simulink model "Vjezba2"  (R2023b)
settings: Solver=ode1  StartTime=0.0  StopTime=simulationTime  FixedStep=sampleTime  RelTol=1e-3  EnableMultiTasking=on
InitFcn:
  | cd(fileparts(which(gcs)))
  | 
  | run ./InitModel.m;
StopFcn:
  | run ./DrawPath.m;
values from neighbouring files (symbols this model uses):
  sampleTime = 1e-2    (= 0.01)    [InitModel.m]
  SWA = 3    [InitModel.m]
  vx0 = 200    [InitModel.m]
undefined symbols (not defined in the file or in its folder): vehicleData
libraries: simulink_extras x1
settings Model: Creator=arikera  LastModifiedBy=lvuke
settings SolverCC: AlgebraicLoopSolver=TrustRegion
settings DataIOCC: LimitDataPoints=on  SaveFormat=Array  SignalLoggingSaveFormat=ModelDataLogs  ReturnWorkspaceOutputs=off
settings OptimizationCC: ExpressionDepthLimit=2147483647  LifeSpan=inf
settings DebuggingCC: UnderspecifiedInitializationDetection=Classic  MergeDetectMultiDrivingBlocksExec=none  SolverPrmCheckMsg=warning  FcnCallInpInsideContextMsg=warning  UnconnectedInputMsg=warning  UnconnectedOutputMsg=warning  UnconnectedLineMsg=warning  AllowSymbolicDim=off  StateNameClashWarn=warning  SFUnexpectedBacktrackingDiag=warning  SFNoUnconditionalDefaultTransitionDiag=warning  SFExecutionAtInitializationDiag=none  ArithmeticOperatorsInVariantConditions=warning
settings HardwareCC: ProdBitPerPointer=32  ProdBitPerSizeT=32  ProdBitPerPtrDiffT=32  ProdLargestAtomicFloat=None  ProdIntDivRoundTo=Undefined  ProdEndianess=Unspecified  ProdWordSize=32  ProdHWDeviceType=32-bit Generic
settings ModelReferenceCC: EnableRefExpFcnMdlSchedulingChecks=on  PropagateSignalLabelsOutOfModel=off
settings SFSimCC: SimUseLocalCustomCode=off  CustomCodeUndefinedFunction=UseInterfaceOnly
settings RTWCC: RTWUseLocalCustomCode=off
settings CodeAppCC: StateflowObjectComments=on
settings GRTTargetCC: TargetLangStandard=C89/C90 (ANSI)  CombineOutputUpdateFcns=off  GRTInterface=on
settings ConfigComp: CovMetricSettings=dw  CovSaveCumulativeToWorkspaceVar=on  CovSaveSingleToWorkspaceVar=on  CovExternalEMLEnable=off  CovSFcnEnable=off

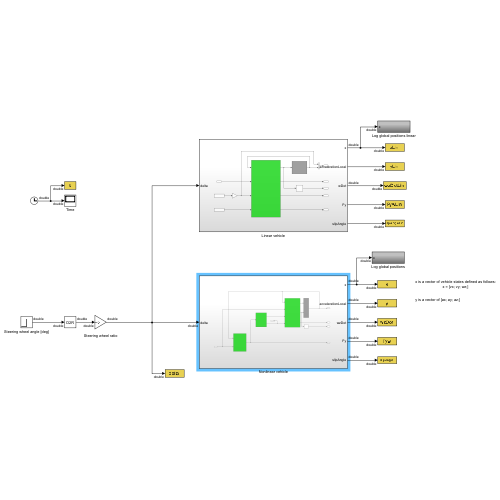
[thumbnail: Simulink's stored preview of the top-level diagram]
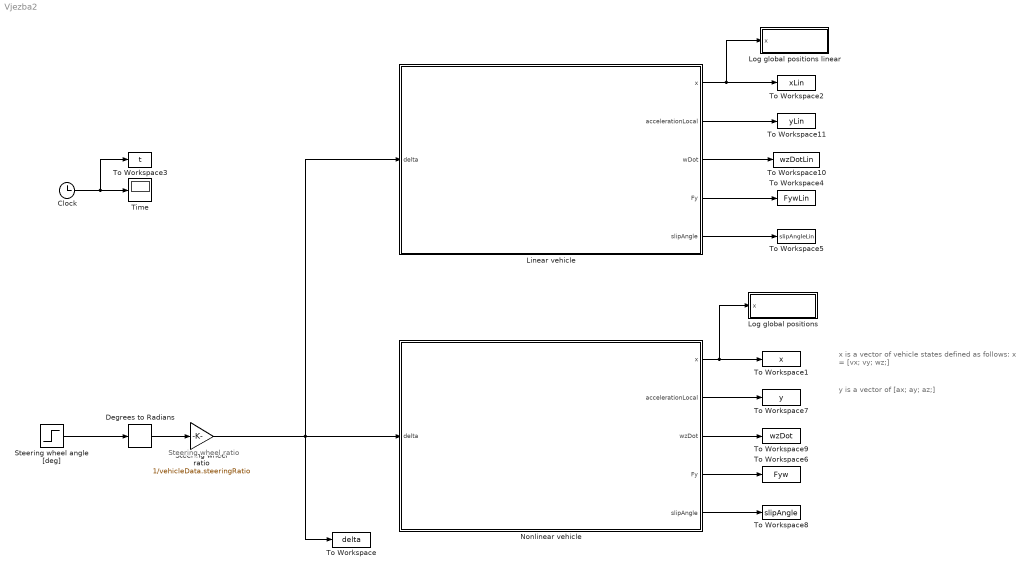
== system Vjezba2 ==
  note: Steering wheel ratio
  note: x is a vector of vehicle states defined as follows:
      | x = [vx; vy; wz;]
  note: y is a vector of [ax; ay; az;]
  Clock : Clock
  Degrees to Radians : simulink_extras/Transformations/Degrees to Radians
  Linear vehicle : Subsystem
  Log global positions : Subsystem
  Log global positions linear : Subsystem
  Nonlinear vehicle : Subsystem
  Steering wheel angle [deg] : Step  Time=3  After=SWA  SampleTime=0
  Steering wheel ratio : Gain  Gain=1/vehicleData.steeringRatio
  Time : Display
  To Workspace : ToWorkspace  VariableName=delta  SampleTime=sampleTime
  To Workspace1 : ToWorkspace  VariableName=x  SampleTime=sampleTime
  To Workspace10 : ToWorkspace  VariableName=wzDotLin  SampleTime=sampleTime
  To Workspace11 : ToWorkspace  VariableName=yLin  SampleTime=sampleTime
  To Workspace2 : ToWorkspace  VariableName=xLin  SampleTime=sampleTime
  To Workspace3 : ToWorkspace  VariableName=t  SampleTime=sampleTime
  To Workspace4 : ToWorkspace  VariableName=FywLin  SampleTime=sampleTime
  To Workspace5 : ToWorkspace  VariableName=slipAngleLin  SampleTime=sampleTime
  To Workspace6 : ToWorkspace  VariableName=Fyw  SampleTime=sampleTime
  To Workspace7 : ToWorkspace  VariableName=y  SampleTime=sampleTime
  To Workspace8 : ToWorkspace  VariableName=slipAngle  SampleTime=sampleTime
  To Workspace9 : ToWorkspace  VariableName=wzDot  SampleTime=sampleTime
  wires:
  Clock/1 -> To Workspace3/1, Time/1
  Steering wheel angle [deg]/1 -> Degrees to Radians/1
  Nonlinear vehicle/1(x) -> Log global positions/1(x), To Workspace1/1
  Nonlinear vehicle/2(accelerationLocal) -> To Workspace7/1
  Nonlinear vehicle/3(wzDot) -> To Workspace9/1
  Nonlinear vehicle/4(Fy) -> To Workspace6/1
  Nonlinear vehicle/5(slipAngle) -> To Workspace8/1
  Linear vehicle/1(x) -> Log global positions linear/1(x), To Workspace2/1
  Linear vehicle/3(wDot) -> To Workspace10/1
  Steering wheel ratio/1 -> Linear vehicle/1(delta), To Workspace/1, Nonlinear vehicle/1(delta)
  Linear vehicle/2(accelerationLocal) -> To Workspace11/1
  Degrees to Radians/1 -> Steering wheel ratio/1
  Linear vehicle/4(Fy) -> To Workspace4/1
  Linear vehicle/5(slipAngle) -> To Workspace5/1

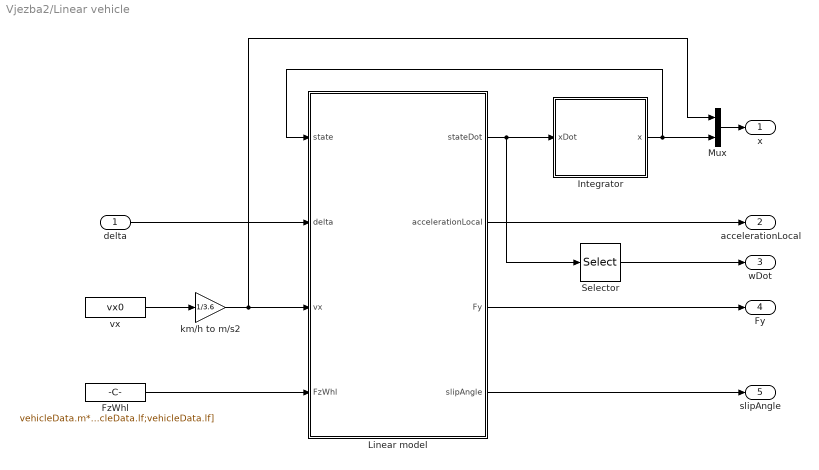
== system Vjezba2/Linear vehicle ==
  delta : Inport
  FzWhl : Constant  Value=vehicleData.m*vehicleData.g/(2*vehicleData.L)*[vehicleData.lr;vehicleData.lr;vehicleData.lf;vehicleData.lf]  SampleTime=0
  Integrator : Subsystem
  Linear model : MATLAB Function  TreatAsAtomicUnit=on
  Mux : Mux  Inputs=2
  Selector : Selector  InputPortWidth=2  IndexOptions=Index vector (dialog)  Indices=[2]  OutputSizes=1
  km/h to m/s2 : Gain  Gain=1/3.6
  vx : Constant  Value=vx0  SampleTime=0
  x : Outport  VectorParamsAs1DForOutWhenUnconnected=off
  accelerationLocal : Outport  Port=2
  wDot : Outport  Port=3  VectorParamsAs1DForOutWhenUnconnected=off
  Fy : Outport  Port=4  VectorParamsAs1DForOutWhenUnconnected=off
  slipAngle : Outport  Port=5  VectorParamsAs1DForOutWhenUnconnected=off
  wires:
  FzWhl/1 -> Linear model/4(FzWhl)
  Linear model/1(stateDot) -> Selector/1, Integrator/1(xDot)
  Integrator/1(x) -> Mux/2, Linear model/1(state)
  delta/1 -> Linear model/2(delta)
  Selector/1 -> wDot/1
  Mux/1 -> x/1
  vx/1 -> km/h to m/s2/1
  km/h to m/s2/1 -> Mux/1, Linear model/3(vx)
  Linear model/2(accelerationLocal) -> accelerationLocal/1
  Linear model/4(slipAngle) -> slipAngle/1
  Linear model/3(Fy) -> Fy/1

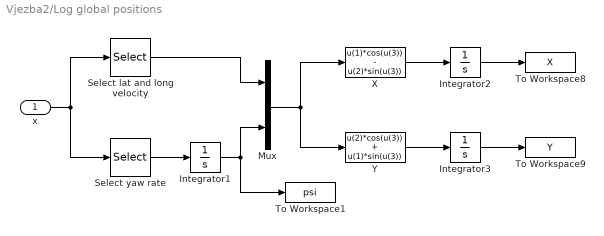
== system Vjezba2/Log global positions ==
  x : Inport
  Integrator1 : Integrator
  Integrator2 : Integrator
  Integrator3 : Integrator
  Mux : Mux  Inputs=2
  Select yaw rate : Selector  InputPortWidth=3  IndexOptions=Index vector (dialog)  Indices=3  OutputSizes=1
  Select lat and long velocity : Selector  InputPortWidth=3  IndexOptions=Index vector (dialog)  Indices=[1 2]  OutputSizes=1
  To Workspace1 : ToWorkspace  VariableName=psi  SampleTime=sampleTime
  To Workspace8 : ToWorkspace  VariableName=X  SampleTime=sampleTime
  To Workspace9 : ToWorkspace  VariableName=Y  SampleTime=sampleTime
  X : Fcn  Expr=u(1)*cos(u(3)) - u(2)*sin(u(3))
  Y : Fcn  Expr=u(2)*cos(u(3)) + u(1)*sin(u(3))
  wires:
  Select yaw rate/1 -> Integrator1/1
  Select lat and long velocity/1 -> Mux/1
  Integrator1/1 -> Mux/2, To Workspace1/1
  Mux/1 -> X/1, Y/1
  X/1 -> Integrator2/1
  Y/1 -> Integrator3/1
  x/1 -> Select yaw rate/1, Select lat and long velocity/1
  Integrator2/1 -> To Workspace8/1
  Integrator3/1 -> To Workspace9/1

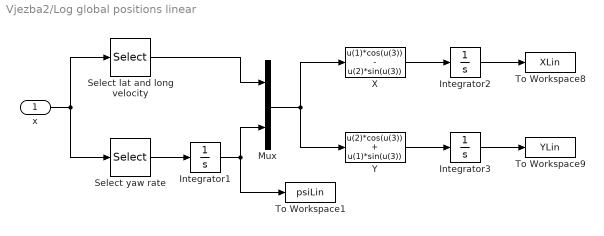
== system Vjezba2/Log global positions linear ==
  x : Inport
  Integrator1 : Integrator
  Integrator2 : Integrator
  Integrator3 : Integrator
  Mux : Mux  Inputs=2
  Select yaw rate : Selector  InputPortWidth=3  IndexOptions=Index vector (dialog)  Indices=3  OutputSizes=1
  Select lat and long velocity : Selector  InputPortWidth=3  IndexOptions=Index vector (dialog)  Indices=[1 2]  OutputSizes=1
  To Workspace1 : ToWorkspace  VariableName=psiLin  SampleTime=sampleTime
  To Workspace8 : ToWorkspace  VariableName=XLin  SampleTime=sampleTime
  To Workspace9 : ToWorkspace  VariableName=YLin  SampleTime=sampleTime
  X : Fcn  Expr=u(1)*cos(u(3)) - u(2)*sin(u(3))
  Y : Fcn  Expr=u(2)*cos(u(3)) + u(1)*sin(u(3))
  wires:
  Select yaw rate/1 -> Integrator1/1
  Select lat and long velocity/1 -> Mux/1
  Integrator1/1 -> Mux/2, To Workspace1/1
  Mux/1 -> X/1, Y/1
  X/1 -> Integrator2/1
  Y/1 -> Integrator3/1
  x/1 -> Select yaw rate/1, Select lat and long velocity/1
  Integrator2/1 -> To Workspace8/1
  Integrator3/1 -> To Workspace9/1

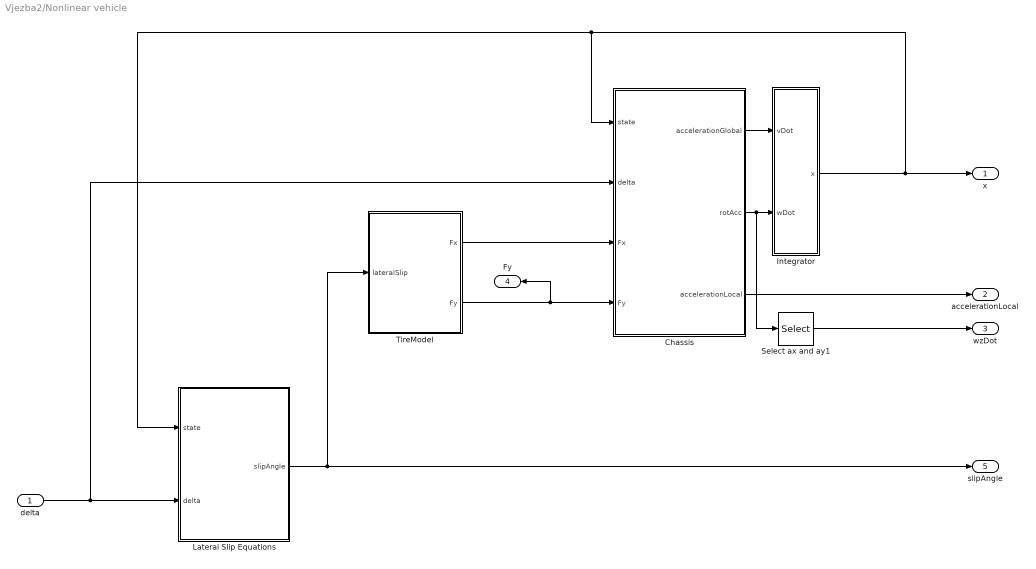
== system Vjezba2/Nonlinear vehicle ==
  delta : Inport
  Chassis : MATLAB Function  TreatAsAtomicUnit=on
  Integrator : Subsystem
  Lateral Slip Equations : MATLAB Function  TreatAsAtomicUnit=on
  Select ax and ay1 : Selector  InputPortWidth=3  IndexOptions=Index vector (dialog)  Indices=[3]  OutputSizes=1
  TireModel : Subsystem
  x : Outport
  accelerationLocal : Outport  Port=2
  wzDot : Outport  Port=3
  Fy : Outport  Port=4
  slipAngle : Outport  Port=5
  wires:
  Chassis/2(rotAcc) -> Select ax and ay1/1, Integrator/2(wDot)
  Chassis/1(accelerationGlobal) -> Integrator/1(vDot)
  delta/1 -> Lateral Slip Equations/2(delta), Chassis/2(delta)
  TireModel/2(Fy) -> Fy/1, Chassis/4(Fy)
  TireModel/1(Fx) -> Chassis/3(Fx)
  Lateral Slip Equations/1(slipAngle) -> slipAngle/1, TireModel/1(lateralSlip)
  Chassis/3(accelerationLocal) -> accelerationLocal/1
  Integrator/1(x) -> Chassis/1(state), Lateral Slip Equations/1(state), x/1
  Select ax and ay1/1 -> wzDot/1

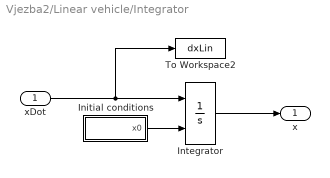
== system Vjezba2/Linear vehicle/Integrator ==
  xDot : Inport
  Initial conditions : Subsystem  mask(x0){v0=0, r0=0}
      mask prompts: v0 "Lateral velocity [km/h]"; r0 "Yaw rate [deg/s]"
      mask help: Initial conditions for the simulation
      mask Help:
      | Sets the initial condition for the simulation.
      | 
      | This is a rather simple block that has been made for assignments in the Vehicle Dynamics course (MMF062) at Chalmers since most students enrolled in this course have no prior experience in Simulink.
      | 
      | This block is equivalent to a constant source block with the vector '[u0, v0, r0, ax0, ay0, rDot0]' as the input, where the parameters are as follows:
      | 
      | u0  - Initial longitudinal velocity
      | v0  - Initial lateral velocity
      | r0  - Initial yaw rate
      | 
      | All the parameters are in SI units.
  Integrator : Integrator  InitialConditionSource=external
  To Workspace2 : ToWorkspace  VariableName=dxLin  SampleTime=sampleTime
  x : Outport  VectorParamsAs1DForOutWhenUnconnected=off
  wires:
  Initial conditions/1(x0) -> Integrator/2
  Integrator/1 -> x/1
  xDot/1 -> To Workspace2/1, Integrator/1

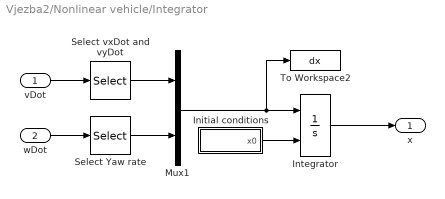
== system Vjezba2/Nonlinear vehicle/Integrator ==
  vDot : Inport
  wDot : Inport  Port=2
  Initial conditions : Subsystem  mask(x0){u0=vx0, v0=0, r0=0}
      mask prompts: u0 "Longitudinal velocity [km/h]"; v0 "Lateral velocity [km/h]"; r0 "Yaw rate [deg/s]"
      mask help: Initial conditions for the simulation
      mask Help:
      | Sets the initial condition for the simulation.
      | 
      | This is a rather simple block that has been made for assignments in the Vehicle Dynamics course (MMF062) at Chalmers since most students enrolled in this course have no prior experience in Simulink.
      | 
      | This block is equivalent to a constant source block with the vector '[u0, v0, r0, ax0, ay0, rDot0]' as the input, where the parameters are as follows:
      | 
      | u0  - Initial longitudinal velocity
      | v0  - Initial lateral velocity
      | r0  - Initial yaw rate
      | 
      | All the parameters are in SI units.
  Integrator : Integrator  InitialConditionSource=external
  Mux1 : Mux  Inputs=2
  Select Yaw rate : Selector  InputPortWidth=3  IndexOptions=Index vector (dialog)  Indices=[3]  OutputSizes=1
  Select vxDot and vyDot : Selector  InputPortWidth=3  IndexOptions=Index vector (dialog)  Indices=[1 2]  OutputSizes=1
  To Workspace2 : ToWorkspace  VariableName=dx  SampleTime=sampleTime
  x : Outport  VectorParamsAs1DForOutWhenUnconnected=off
  wires:
  Select Yaw rate/1 -> Mux1/2
  wDot/1 -> Select Yaw rate/1
  Select vxDot and vyDot/1 -> Mux1/1
  vDot/1 -> Select vxDot and vyDot/1
  Mux1/1 -> To Workspace2/1, Integrator/1
  Initial conditions/1(x0) -> Integrator/2
  Integrator/1 -> x/1

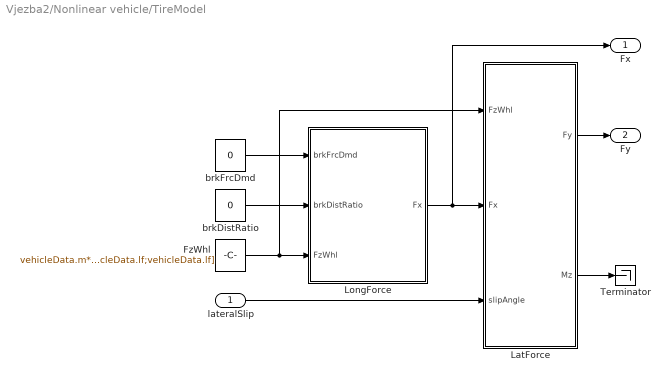
== system Vjezba2/Nonlinear vehicle/TireModel ==
  lateralSlip : Inport
  FzWhl : Constant  Value=vehicleData.m*vehicleData.g/(2*vehicleData.L)*[vehicleData.lr;vehicleData.lr;vehicleData.lf;vehicleData.lf]  SampleTime=0
  LatForce : MATLAB Function  TreatAsAtomicUnit=on
  LongForce : MATLAB Function  TreatAsAtomicUnit=on
  Terminator : Terminator
  brkDistRatio : Constant  Value=0  SampleTime=0
  brkFrcDmd : Constant  Value=0  SampleTime=0
  Fx : Outport  VectorParamsAs1DForOutWhenUnconnected=off
  Fy : Outport  Port=2  VectorParamsAs1DForOutWhenUnconnected=off
  wires:
  LongForce/1(Fx) -> LatForce/2(Fx), Fx/1
  LatForce/1(Fy) -> Fy/1
  LatForce/2(Mz) -> Terminator/1
  lateralSlip/1 -> LatForce/3(slipAngle)
  FzWhl/1 -> LatForce/1(FzWhl), LongForce/3(FzWhl)
  brkDistRatio/1 -> LongForce/2(brkDistRatio)
  brkFrcDmd/1 -> LongForce/1(brkFrcDmd)

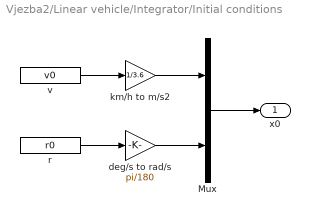
== system Vjezba2/Linear vehicle/Integrator/Initial conditions ==
  Mux : Mux  Inputs=2
  deg/s to rad/s : Gain  Gain=pi/180
  km/h to m/s2 : Gain  Gain=1/3.6
  r : Constant  Value=r0
  v : Constant  Value=v0
  x0 : Outport  VectorParamsAs1DForOutWhenUnconnected=off
  wires:
  Mux/1 -> x0/1
  v/1 -> km/h to m/s2/1
  r/1 -> deg/s to rad/s/1
  km/h to m/s2/1 -> Mux/1
  deg/s to rad/s/1 -> Mux/2

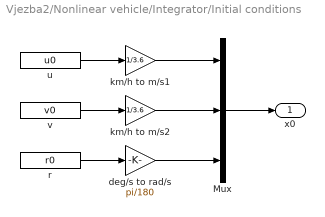
== system Vjezba2/Nonlinear vehicle/Integrator/Initial conditions ==
  Mux : Mux  Inputs=3
  deg/s to rad/s : Gain  Gain=pi/180
  km/h to m/s1 : Gain  Gain=1/3.6
  km/h to m/s2 : Gain  Gain=1/3.6
  r : Constant  Value=r0
  u : Constant  Value=u0
  v : Constant  Value=v0
  x0 : Outport  VectorParamsAs1DForOutWhenUnconnected=off
  wires:
  Mux/1 -> x0/1
  u/1 -> km/h to m/s1/1
  v/1 -> km/h to m/s2/1
  r/1 -> deg/s to rad/s/1
  km/h to m/s1/1 -> Mux/1
  km/h to m/s2/1 -> Mux/2
  deg/s to rad/s/1 -> Mux/3

== matlab function Vjezba2/Nonlinear vehicle/TireModel/LongForce ==
  data: brkFrcDmd input; brkDistRatio input; FzWhl input; Fx output
 function Fx  = LongForce(brkFrcDmd,brkDistRatio,FzWhl)
    % Inputs:
    %   FzWhl        - Normal load on tires [N]
    %   brkDistRatio - Front to total brake distribution ratio [-]
    %   brkFrcDmd    - Total brake force demand
    % Outputs:
    %   Fx           - A [2x1] vector with axle longitudinal forces [N]
    
    %%========================DO NOT CHANGE THIS=============================%%
    mu          = 0.8;                                   % Limiting friction coefficient
    FzWhl       = max(FzWhl,[0;0;0;0]);                  % Make sure normal load on wheel does not become negative
    FzFrontAxle = FzWhl(1)+FzWhl(2);                     % Front axle normal load
    FzRearAxle  = FzWhl(3)+FzWhl(4);                     % Rear axle normal load

    %%=======================================================================%%
    % Longitudinal Force
    brkFrcFront = brkDistRatio*brkFrcDmd;                % Braking force on front axle
    brkFrcRear  = brkFrcDmd-brkFrcFront;                 % Braking force on rear axle
    FxFront     = -min(mu*FzFrontAxle,abs(brkFrcFront)); % Limit maximum value
    FxRear      = -min(mu*FzRearAxle,abs(brkFrcRear));   % Limit maximum value
    Fx          = [FxFront;FxRear];
    %%=======================================================================%%
end

== matlab function Vjezba2/Nonlinear vehicle/TireModel/LatForce ==
  data: FzWhl input; Fx input; slipAngle input; Fy output; vehicleData parameter; Mz output
function [Fy,Mz]  = LatForce(FzWhl,Fx,slipAngle,vehicleData)
    % Inputs:
    %   FzWhl      - Normal load on tires [N]
    %   Fx         - Longitudinal force vector [N]
    %   slipAngle  - Slip angle vector [rad]
    % Outputs:
    %   Fy         - A [2x1] vector with axle lateral forces [N]
    %   Mz         - Dummy value for StrWhlTrq [Nm]
    %
    %%=======================================================================%%
    c0          = vehicleData.c0;                       % Tyre stiffness parameter
    c1          = vehicleData.c1;                       % Tyre stiffness parameter
    mu          = 0.8;

    FzWhl       = max(FzWhl,[0;0;0;0]);                 % Limit minimum value
    FzFrontAxle = FzWhl(1)+FzWhl(2);                    % Front axle normal load
    FzRearAxle  = FzWhl(3)+FzWhl(4);                    % Rear axle normal load
    FzAxle      = [FzFrontAxle;FzRearAxle];
    %%=======================================================================%%
    
    % Axle stiffness calculation (keep in mind that the tyre data is for one
    % wheel and not an axle)
    maxLatForce = [0;0];
    
    % Fx could have been limited when it is calculated
    if (Fx(1)^2>=(mu*FzFrontAxle)^2)
        Cf             = 1e-3;                             % Solving the numerical problems
        maxLatForce(1) = 0;
    else
        %%=======================================================================%%
        Cf =  c0*(FzWhl(1)+FzWhl(2)) + c1*(FzWhl(1)^2+FzWhl(2)^2);  % Front cornering stiffness
        maxLatForce(1) = sqrt((mu*FzAxle(1))^2-Fx(1)^2);   % Friction circle
    end
    
    if (Fx(2)^2>=(mu*FzRearAxle)^2)
        Cr             = 1e-3;                             % Solving the numerical problems
        maxLatForce(2) = 0;
    else
        Cr = c0*(FzWhl(3)+FzWhl(4)) + c1*(FzWhl(3)^2+FzWhl(4)^2);  % Rear cornering stiffness        
        maxLatForce(2) = sqrt((mu*FzAxle(2))^2-Fx(2)^2);   % Friction circle
    end
    
    % Lateral force
    CAxle = [Cf;Cr];
    Fy    =  -CAxle .* slipAngle;
    
    %%=======================================================================%%
    Fy    = min(maxLatForce,abs(Fy)).*sign(Fy);            % Saturation of Fy to sqrt(Fz^2-Fx^2)
    %%=======================================================================%%
    % Self-aligning moment
    A  = -0.001;
    C  = 0.4;
    Mz = A*Fy(1)*C;
    %%=======================================================================%%
end

== matlab function Vjezba2/Linear vehicle/Linear model ==
  data: state input; delta input; vx input; FzWhl input; stateDot output; vehicleData parameter; accelerationLocal output; Fy output; slipAngle output
function [stateDot,accelerationLocal,Fy,slipAngle] = LinearModel(state, delta, vx, FzWhl, vehicleData)
    % Inputs:
    %   state  - state vector
    %   delta  - steering wheel angle [rad]
    %   vx     - longitudinal velocity
    %   FzWhl  - Normal load on tires [N]
    % Outputs:
    %   stateDot            - global vehicle acceleration
    %                         [vyDot; wzDot]
    %   accelerationLocal   - local vehicle acceleration 
    %                         [ax; ay; az]

    % ----- Parameters -----
    %%========================DO NOT CHANGE THIS=============================%%
    c0        = vehicleData.c0;           % Tyre stiffness parameter
    c1        = vehicleData.c1;           % Tyre stiffness parameter
    m         = vehicleData.m;            % Mass of the vehicle
    J         = vehicleData.J;            % Yaw inertia of the vehicle
    lf        = vehicleData.lf;           % Distance of CoG from front axle
    lr        = vehicleData.lr;           % Distance of CoG from rear axle
    
    FzWhl       = max(FzWhl,[0;0;0;0]);                 % Limit minimum value
    
    % Axle stiffness calculation (keep in mind that the tyre data is for one
    % wheel and not an axle)
    Cf = c0*(FzWhl(1)+FzWhl(2)) + c1*(FzWhl(1)^2+FzWhl(2)^2);
    Cr = c0*(FzWhl(3)+FzWhl(4)) + c1*(FzWhl(3)^2+FzWhl(4)^2); 

    % State vector
    vy        = state(1);
    wz        = state(2);
    
    %%===========================FOR TASK 2.1================================%%
    % Matrices of the system
   
    % Elements of the A matrix
    A = zeros(2,2);
    A(1,1) = -(Cf + Cr) / (m * vx);
    A(1,2) = (lf * Cf - lr * Cr) / (m * vx) - vx;
    A(2,1) = (lf * Cf - lr * Cr) / (J * vx);
    A(2,2) = (lf^2 * Cf + lr^2 * Cr) / (J * vx);
    
    % Elements of the B matrix
    B = zeros(2,1);
    B(1,1) = Cf / m;
    B(2,1) = lf * Cf / J;
    %%========================DO NOT CHANGE THIS=============================%%
    stateDot = A*state + B*delta;
    %%=======================================================================%%
    % Accelerations
    ax                 = 0; 
    ay                 = stateDot(1)+wz*vx;
    az                 = 0;
    accelerationLocal  = [ax;ay;az];

    % Slip angles
    alphaf    = (vy + wz*lf)/vx - delta;
    alphar    = (vy - wz*lf)/vx;
    slipAngle = [alphaf;alphar];

    % Lateral forces
    Fyf = -Cf*alphaf;
    Fyr = -Cr*alphar;
    Fy  = [Fyf;Fyr];
    %%=======================================================================%%
end

== matlab function Vjezba2/Nonlinear vehicle/Chassis ==
  data: state input; accelerationGlobal output; rotAcc output; delta input; Fx input; Fy input; accelerationLocal output; vehicleData parameter
function [accelerationGlobal,rotAcc,accelerationLocal] = VehDynModel(state,delta,Fx,Fy,vehicleData)
    % Inputs:
    %   state  - state vector
    %   delta  - steering wheel angle [rad]
    %   Fx     - Vector of forces from the wheels in x-direction
    %   Fy     - Vector of forces from the wheels in y-direction
    % Outputs: 
    %   accelerationGlobal  - global vehicle acceleration
    %                         [vxDot; vyDot; vzDot]
    %   rotAcc              - vector of vehicle rotational accelerations
    %                         [wx; wy; wz]
    %   accelerationLocal   - local vehicle acceleration 
    %                         [ax; ay; az]
    %
    % ----- Parameters -----
    %%========================DO NOT CHANGE THIS=============================%%
    m         = vehicleData.m;            % Mass of vehicle
    J         = vehicleData.J;
    lf        = vehicleData.lf;           % Distance of CoG from front axle
    lr        = vehicleData.lr;           % Distance of CoG from rear axle

    % State vector
    vx        = state(1);
    vy        = state(2);
    wz        = state(3);
    
    %%===========================FOR TASK 2.2================================%%
    % Equations of motion
    vxDot     = (Fx(2) + Fx(1)*cos(delta) - Fy(1)*sin(delta) + m*vy*wz)/m;  % Derivative of longtidunial velocity
    vyDot     = (Fy(2) + Fy(1)*cos(delta) + Fx(1)*sin(delta) - m*vx*wz)/m;  % Derivative of lateral velocity
    wzDot     = (Fy(1)*cos(delta)*lf - Fy(2)*lr + Fx(1)*sin(delta)*lf)/J;  % Derivative of yaw rotational velocity
    
    %%========================DO NOT CHANGE THIS=============================%%
    vzDot     = 0;
    wxDot     = 0;
    wyDot     = 0;
      

    % Accelerations
    accelerationGlobal = [vxDot;vyDot;vzDot];
    ax                 = vxDot-wz*vy; 
    ay                 = vyDot+wz*vx;
    az                 = 0;
    accelerationLocal  = [ax;ay;az];

    % Rotational accelerations
    rotAcc             = [wxDot;wyDot;wzDot];
    %%=======================================================================%%
end

% end of file

== matlab function Vjezba2/Nonlinear vehicle/Lateral Slip Equations ==
  data: state input; slipAngle output; delta input; vehicleData parameter
function slipAngle   = LateralSlip(state,delta,vehicleData) 
    % Inputs:
    %   state     - State vector
    %   delta     - steering wheel angle [rad]
    % Outputs:
    %   slipangle - A [2x1] vector containing the slipratio(0-1) for each axle [-]
    %
    %%========================DO NOT CHANGE THIS=============================%%
    % ----- Parameters -----
    % State vector
    vx = state(1);
    vy = state(2);
    wz = state(3);
    lf = vehicleData.lf;           % Distance of CoG from front axle
    lr = vehicleData.lr;           % Distance of CoG from rear axle
    % Preventing vx from being zero 
    vx = max(abs(vx),3);

    %%===========================FOR TASK 2.2================================%%
    % Slip equations
    alphaf    = (-vx*delta + vy + wz*lf)/(vx + (vy + wz*lf)*delta);  
    %  Front lateral tire slip 
    alphar    = (vy - wz*lr)/vx;   %  Rear lateral tire slip
    
    slipAngle = [alphaf; alphar];  % Slip angle vector
    %%=======================================================================%%

end

% end of file
